simulink model "steering"  (R2015b)
settings: Solver=VariableStepAuto  StartTime=0.0  StopTime=20  RelTol=1e-3
settings Model: Creator=Thomas  LastModifiedBy=Mads

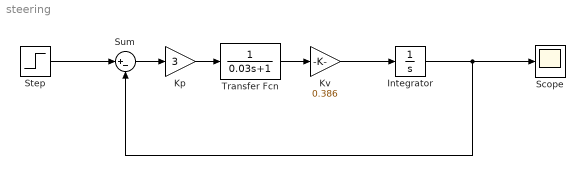
== system steering ==
  Integrator : Integrator
  Kp : Gain  Gain=3
  Kv : Gain  Gain=0.386
  Scope : Scope
  Step : Step  Time=10  Before=5  After=45  SampleTime=0
  Sum : Sum  Inputs=|+-
  Transfer Fcn : TransferFcn  Denominator=[0.03 1]
  wires:
  Kv/1 -> Integrator/1
  Sum/1 -> Kp/1
  Step/1 -> Sum/1
  Kp/1 -> Transfer Fcn/1
  Transfer Fcn/1 -> Kv/1
  Integrator/1 -> Sum/2, Scope/1
